simulink model "s_aero2_2dof_pd"  (R2021a)
settings: Solver=ode4  StartTime=0.0  StopTime=30  FixedStep=0.002  RelTol=1e-3
values from neighbouring files (symbols this model uses):
  Dp = 0.00199    [aero2_parameters_id.m]
  Dt = 0.16743    [aero2_parameters.m]
  Dy = 0.00192    [aero2_parameters_id.m]
  Jp = 23188500.45 / 1000 * 0.001^2    (= 0.02318850045)    [aero2_parameters.m]
  Jy = 23810415.95 / 1000 * 0.001^2    (= 0.02381041595)    [aero2_parameters.m]
  Kpp = 0.00321    [aero2_parameters_id.m]
  Kpy = 0.00137    [aero2_parameters_id.m]
  Ksp = 0.00744    [aero2_parameters_id.m]
  Kyp = -0.00319    [aero2_parameters_id.m]
  Kyy = 0.00610    (= 0.0061)    [aero2_parameters_id.m]
undefined symbols (not defined in the file or in its folder): kp_p, kp_y
libraries: simulink_extras x4, quarc_library x2
settings Model: Creator=MLevis  LastModifiedBy=mbohra
settings SolverCC: AlgebraicLoopSolver=TrustRegion
settings DataIOCC: ReturnWorkspaceOutputs=off
settings DebuggingCC: SFMachineParentedDataDiag=warning

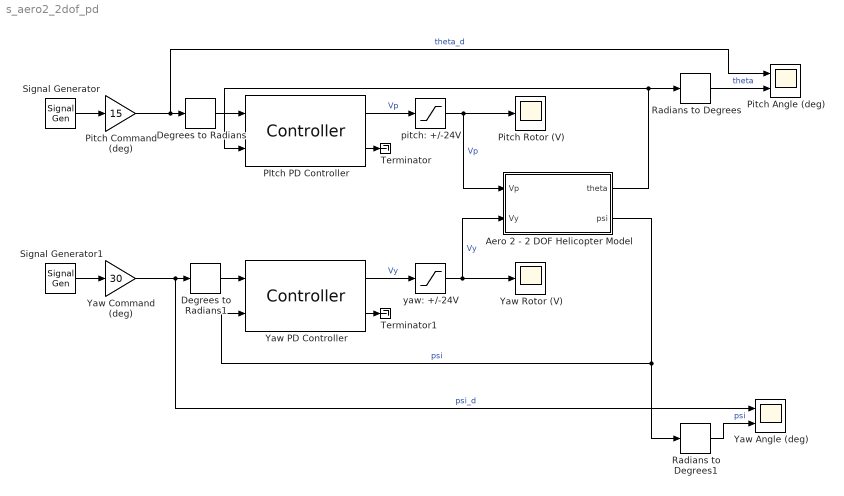
== system s_aero2_2dof_pd ==
  Aero 2 - 2 DOF Helicopter Model : Subsystem
  Degrees to Radians : simulink_extras/Transformations/Degrees to Radians
  Degrees to Radians1 : simulink_extras/Transformations/Degrees to Radians
  PItch PD Controller : quarc_library/Continuous/Controller  ctrl_type=Proportional-Integral-Velocity (PIV)  param_src=Specify via dialog  Kp=kp_p  Ki=0  Kd=0  Kv=kd_p  Ka=0  Wn=100
      settings: SourceProductName=QUARC Targets
  Pitch Angle (deg) : Scope  NumInputPorts=2
  Pitch Command (deg) : Gain  Gain=15
  Pitch Rotor (V) : Scope
  Radians to Degrees : simulink_extras/Transformations/Radians to Degrees
  Radians to Degrees1 : simulink_extras/Transformations/Radians to Degrees
  Signal Generator : SignalGenerator  WaveForm=square  Frequency=0.05
  Signal Generator1 : SignalGenerator  WaveForm=square  Frequency=0.04
  Terminator : Terminator
  Terminator1 : Terminator
  Yaw Angle (deg) : Scope  NumInputPorts=2
  Yaw Command (deg) : Gain  Gain=30
  Yaw PD Controller : quarc_library/Continuous/Controller  ctrl_type=Proportional-Integral-Velocity (PIV)  param_src=Specify via dialog  Kp=kp_y  Ki=0  Kd=0  Kv=kd_y  Ka=0  Wn=100
      settings: SourceProductName=QUARC Targets
  Yaw Rotor (V) : Scope
  pitch: +/-24V : Saturate  UpperLimit=24  LowerLimit=-24
  yaw: +/-24V : Saturate  UpperLimit=24  LowerLimit=-24
  wires:
  Pitch Command (deg)/1 -> Pitch Angle (deg)/1, Degrees to Radians/1  "theta_d"
  Yaw Command (deg)/1 -> Yaw Angle (deg)/1, Degrees to Radians1/1  "psi_d"
  yaw: +/-24V/1 -> Aero 2 - 2 DOF Helicopter Model/2(Vy), Yaw Rotor (V)/1  "Vy"
  pitch: +/-24V/1 -> Aero 2 - 2 DOF Helicopter Model/1(Vp), Pitch Rotor (V)/1  "Vp"
  Degrees to Radians1/1 -> Yaw PD Controller/1
  Degrees to Radians/1 -> PItch PD Controller/1
  Radians to Degrees/1 -> Pitch Angle (deg)/2  "theta"
  Radians to Degrees1/1 -> Yaw Angle (deg)/2  "psi"
  Aero 2 - 2 DOF Helicopter Model/2(psi) -> Yaw PD Controller/2, Radians to Degrees1/1  "psi"
  Signal Generator1/1 -> Yaw Command (deg)/1
  Signal Generator/1 -> Pitch Command (deg)/1
  PItch PD Controller/1 -> pitch: +/-24V/1  "Vp"
  Yaw PD Controller/1 -> yaw: +/-24V/1  "Vy"
  Aero 2 - 2 DOF Helicopter Model/1(theta) -> PItch PD Controller/2, Radians to Degrees/1
  PItch PD Controller/2 -> Terminator/1
  Yaw PD Controller/2 -> Terminator1/1

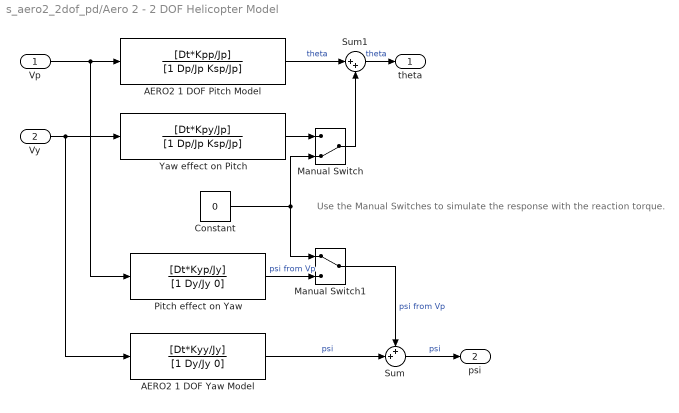
== system s_aero2_2dof_pd/Aero 2 - 2 DOF Helicopter Model ==
  note: Use the Manual Switches to simulate the response with the reaction torque.
  Vp : Inport
  Vy : Inport  Port=2
  AERO2 1 DOF Pitch Model : TransferFcn  Numerator=[Dt*Kpp/Jp]  Denominator=[1 Dp/Jp Ksp/Jp]
  AERO2 1 DOF Yaw Model : TransferFcn  Numerator=[Dt*Kyy/Jy]  Denominator=[1 Dy/Jy 0]
  Constant : Constant  Value=0
  Manual Switch : ManualSwitch  CurrentSetting=0
  Manual Switch1 : ManualSwitch
  Pitch effect on Yaw : TransferFcn  Numerator=[Dt*Kyp/Jy]  Denominator=[1 Dy/Jy 0]
  Sum : Sum  Inputs=++|
  Sum1 : Sum  Inputs=|++
  Yaw effect on Pitch : TransferFcn  Numerator=[Dt*Kpy/Jp]  Denominator=[1 Dp/Jp Ksp/Jp]
  theta : Outport
  psi : Outport  Port=2
  wires:
  AERO2 1 DOF Pitch Model/1 -> Sum1/1  "theta"
  Pitch effect on Yaw/1 -> Manual Switch1/2  "psi from Vp"
  Constant/1 -> Manual Switch1/1, Manual Switch/2
  Manual Switch/1 -> Sum1/2
  Yaw effect on Pitch/1 -> Manual Switch/1
  Vy/1 -> AERO2 1 DOF Yaw Model/1, Yaw effect on Pitch/1
  Vp/1 -> Pitch effect on Yaw/1, AERO2 1 DOF Pitch Model/1
  Sum1/1 -> theta/1  "theta"
  Manual Switch1/1 -> Sum/1  "psi from Vp"
  Sum/1 -> psi/1  "psi"
  AERO2 1 DOF Yaw Model/1 -> Sum/2  "psi"
